simulink model "Q2_Part_a"  (R2015a)
settings: Solver=ode45  StartTime=0.0  StopTime=10.0  RelTol=1e-3
libraries: cstblocks x4
settings Model: Creator=yarde_000  LastModifiedBy=yarde_000

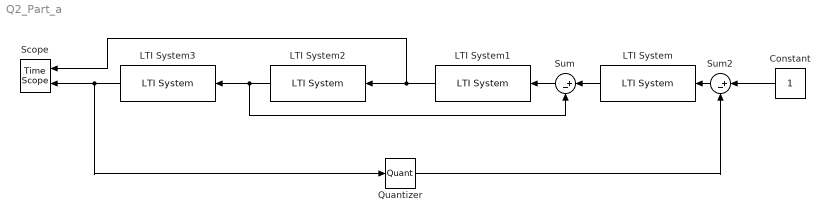
== system Q2_Part_a ==
  Constant : Constant
  LTI System : cstblocks/LTI System  sys=Cp  IC=[]
  LTI System1 : cstblocks/LTI System  sys=Cpi  IC=[]
  LTI System2 : cstblocks/LTI System  sys=P  IC=[]
  LTI System3 : cstblocks/LTI System  sys=tf(1, [1 0])  IC=[]
  Quantizer : Quantizer  QuantizationInterval=enc_res
  Scope : TimeScope  NumInputPorts=2
  Sum : Sum  Inputs=|+-
  Sum2 : Sum  Inputs=|+-
  wires:
  Sum/1 -> LTI System1/1
  LTI System/1 -> Sum/1
  LTI System1/1 -> Scope/1, LTI System2/1
  LTI System2/1 -> Sum/2, LTI System3/1
  LTI System3/1 -> Scope/2, Quantizer/1
  Sum2/1 -> LTI System/1
  Constant/1 -> Sum2/1
  Quantizer/1 -> Sum2/2
